simulink model "Missile_Step_Impulse"  (R2018b)
settings: Solver=ode4  StartTime=0.0  StopTime=7  FixedStep=Step_Size  RelTol=1e-3
InitFcn:
  | clc ;
  | clear all ;
  | close all ;
  | Missile_Data ;
  | Sim_Parameters ;
values from neighbouring files (symbols this model uses):
  ALT = [0.0 1000 2000 3000 4000]    [Sim_Parameters.m]
  Init_Rate = [ 0.0, 0.0, 0.0 ] * UNIT_DEG2RAD    [Sim_Parameters.m]
  Init_Vel = [ 238.0, 0.0, 0.0 ]    [Sim_Parameters.m]
  SOS_Table = [340.268 336.408 332.504  328.553 324.554]    [Sim_Parameters.m]
  UNIT_GRAV = 9.81    [Sim_Parameters.m]
undefined symbols (not defined in the file or in its folder): Alt_Trim, D, Mass, S, Tbl_ALPHAT, Tbl_CL_ALPHAT, Tbl_CL_DEL_R, Tbl_CL_P, Tbl_CM_0, Tbl_CM_DEL_P, Tbl_CM_PHIT, Tbl_CM_Q, Tbl_CN_DEL_Y, Tbl_CN_PHIT, Tbl_CN_R, Tbl_CX_0, Tbl_CX_ALPHAT, Tbl_CX_DEL_EFF, Tbl_CY_DEL_Y, Tbl_CY_PHIT, Tbl_CZ_0, Tbl_CZ_DEL_P, Tbl_CZ_PHIT, Tbl_MACH, XCG, XREF
libraries: simulink_extras x13, aerolibtransform2 x4, UAS_Model_library x4, aerolibasang x3, dspsrcs4 x3, shared6dofsys x1, sharedutil x1, shared6dof x1
settings Model: Creator=e803534  LastModifiedBy=auten
settings OptimizationCC: LifeSpan=inf
settings DebuggingCC: LibraryContextMissingDiagnostic=none  SFUnexpectedBacktrackingDiag=warning  SFNoUnconditionalDefaultTransitionDiag=warning  SFExecutionAtInitializationDiag=none
settings SFSimCC: SimUseLocalCustomCode=off
settings RTWCC: RTWUseLocalCustomCode=off
settings CodeAppCC: StateflowObjectComments=on
settings GRTTargetCC: TargetLangStandard=C89/C90 (ANSI)  GeneratePreprocessorConditionals=Disable all
settings ConfigComp: CovMetricSettings=dw  CovHtmlReporting=on  CovSaveCumulativeToWorkspaceVar=on  CovSaveSingleToWorkspaceVar=on  CovExternalEMLEnable=off

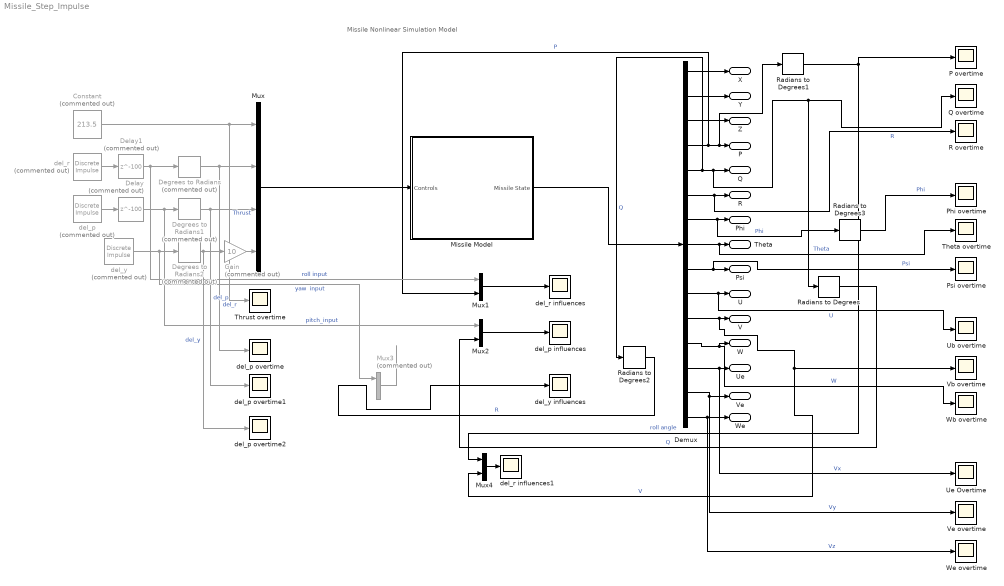
== system Missile_Step_Impulse ==
  note: Missile Nonlinear Simulation Model
  Constant : Constant  Commented=on  Value=213.5  VectorParams1D=off  SampleTime=-1
  Degrees to Radians : simulink_extras/Transformations/Degrees to Radians  Commented=on
  Degrees to Radians1 : simulink_extras/Transformations/Degrees to Radians  Commented=on
  Degrees to Radians2 : simulink_extras/Transformations/Degrees to Radians  Commented=on
  Delay : Delay  Commented=on  DelayLength=100
  Delay1 : Delay  Commented=on  DelayLength=100
  Demux : Demux  Outputs=15
  Gain : Gain  Commented=on  Gain=10
  Missile Model : Subsystem
  Mux : Mux
  Mux1 : Mux  Inputs=2
  Mux2 : Mux  Inputs=2
  Mux3 : Mux  Commented=on  Inputs=3
  Mux4 : Mux  Inputs=2
  P overtime : Scope
  Phi overtime : Scope
  Psi overtime : Scope
  Q overtime : Scope
  R overtime : Scope
  Radians to Degrees{,1..3} (4 alike) : simulink_extras/Transformations/Radians to Degrees
  Theta overtime : Scope
  Thrust overtime : Scope
  Ub overtime : Scope
  Ue Overtime : Scope
  Vb overtime : Scope
  Ve overtime : Scope
  Wb overtime : Scope
  We overtime : Scope
  del_p : dspsrcs4/Discrete  Impulse  Commented=on  Delay=1  SampleTime=0.1  FrameSample=1  OutputFrames=off  dataType=double  isSigned=on  wordLen=16  udDataType=sfix(16)  fracBitsMode=Best precision  numFracBits=15  OutDataTypeStr=double  LastOutDataTypeStr=double
  del_p influences : Scope
  del_p overtime : Scope
  del_p overtime1 : Scope
  del_p overtime2 : Scope
  "del_r " : dspsrcs4/Discrete  Impulse  Commented=on  Delay=1  SampleTime=0.1  FrameSample=1  OutputFrames=off  dataType=double  isSigned=on  wordLen=16  udDataType=sfix(16)  fracBitsMode=Best precision  numFracBits=15  OutDataTypeStr=double  LastOutDataTypeStr=double
  del_r influences : Scope
  del_r influences1 : Scope
  del_y : dspsrcs4/Discrete  Impulse  Commented=on  Delay=1  SampleTime=0.001  FrameSample=1  OutputFrames=off  dataType=double  isSigned=on  wordLen=16  udDataType=sfix(16)  fracBitsMode=Best precision  numFracBits=15  OutDataTypeStr=double  LastOutDataTypeStr=double
  del_y influences : Scope
  X : Outport
  Y : Outport  Port=2
  Z : Outport  Port=3
  P : Outport  Port=4
  Q : Outport  Port=5
  R : Outport  Port=6
  Phi : Outport  Port=7
  Theta : Outport  Port=8
  Psi : Outport  Port=9
  U : Outport  Port=10
  V : Outport  Port=11
  W : Outport  Port=12
  Ue : Outport  Port=13
  Ve : Outport  Port=14
  We : Outport  Port=15
  wires:
  Mux/1 -> Missile Model/1(Controls)
  Demux/11 -> Mux4/2, Vb overtime/1, V/1  "V"
  Demux/4 -> Mux1/2, Radians to Degrees1/1, P/1  "P"
  Demux/10 -> Ub overtime/1, U/1  "U"
  Demux/6 -> R overtime/1, R/1  "R"
  Demux/9 -> Psi overtime/1, Psi/1  "Psi"
  Demux/3 -> Z/1
  Demux/2 -> Y/1
  Demux/12 -> Wb overtime/1, W/1  "W"
  Demux/5 -> Radians to Degrees2/1, Radians to Degrees/1, Q overtime/1, Q/1  "Q"
  Demux/1 -> X/1
  Demux/7 -> Radians to Degrees3/1, Phi/1  "Phi"
  Missile Model/1(Missile State) -> Demux/1
  Degrees to Radians/1 -> del_p overtime/1, Mux/2  "del_r"
  Degrees to Radians1/1 -> Mux/3, del_p overtime1/1  "del_p"
  Degrees to Radians2/1 -> Gain/1, del_p overtime2/1  "del_y"
  Demux/15 -> We overtime/1, We/1  "Vz"
  Demux/14 -> Ve/1, Ve overtime/1  "Vy"
  Demux/13 -> Ue Overtime/1, Ue/1  "Vx"
  Demux/8 -> Theta overtime/1, Theta/1  "Theta"
  "del_r "/1 -> Delay1/1
  del_p/1 -> Delay/1
  Delay/1 -> Degrees to Radians1/1, Mux2/1  "pitch_input"
  Constant/1 -> Thrust overtime/1, Mux/1  "Thrust"
  del_y/1 -> Mux3/1, Degrees to Radians2/1  "yaw  input"
  Delay1/1 -> Mux1/1, Degrees to Radians/1  "roll input"
  Mux1/1 -> del_r influences/1
  Mux2/1 -> del_p influences/1
  Mux3/1 -> ?
  Radians to Degrees1/1 -> P overtime/1, Mux4/1  "roll angle"
  Mux4/1 -> del_r influences1/1
  Radians to Degrees/1 -> Mux2/2  "Q"
  Radians to Degrees2/1 -> del_y influences/1  "R"
  Gain/1 -> Mux/4
  Radians to Degrees3/1 -> Phi overtime/1  "Phi"

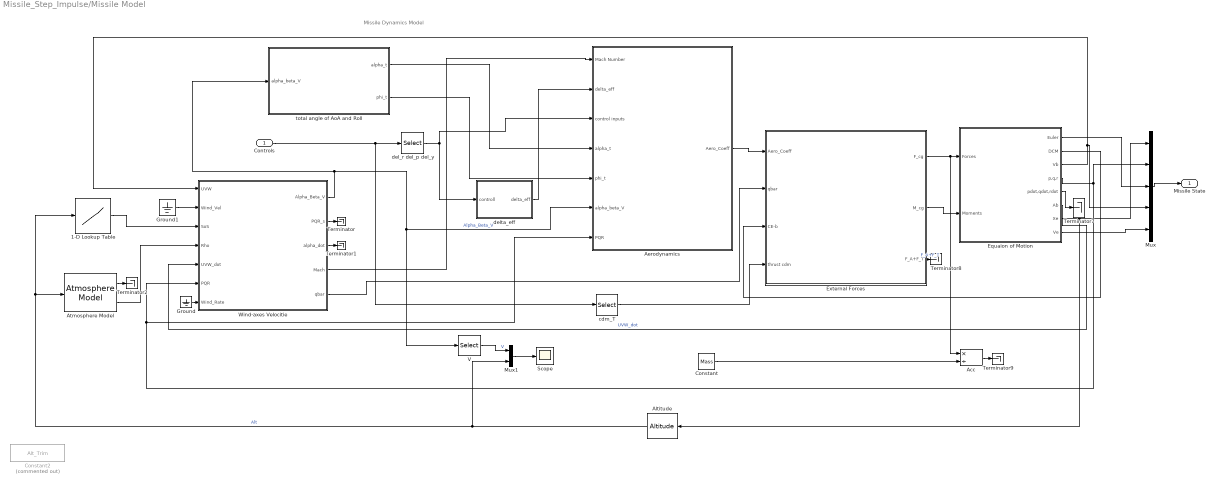
== system Missile_Step_Impulse/Missile Model ==
  note: Missile Dynamics Model
  Controls : Inport
  1-D Lookup Table : Lookup_n-D  NumberOfTableDimensions=1  BreakpointsForDimension1=ALT  Table=SOS_Table  InternalRulePriority=Speed  RndMeth=Simplest  InputSameDT=on
  Acc : Product  Inputs=*/  RndMeth=Zero
  Aerodynamics : Subsystem
  Altitude : UAS_Model_library/Equations of Motion/Altitude  SystemSampleTime=-1
  Atmosphere Model : UAS_Model_library/Envrionment/Atmosphere Model  SystemSampleTime=-1
  Constant : Constant  Value=Mass
  Constant2 : Constant  Commented=on  Value=Alt_Trim
  Equaion of Motion : Subsystem
  External Forces : Subsystem
  Ground : Ground
  Ground1 : Ground
  Mux : Mux  Inputs=5
  Mux1 : Mux  Inputs=2
  Scope : Scope
  Terminator{,1..2,7..9} (6 alike) : Terminator
  V : Selector  InputPortWidth=3  IndexOptions=Index vector (dialog)  Indices=[3]  OutputSizes=1
  Wind-axes Velocitie : Subsystem  AncestorBlock=UAS_Model_library/External Forces/Aerodynamics/Wind-axes Velocitie
  cdm_T : Selector  InputPortWidth=4  IndexOptions=Index vector (dialog)  Indices=[1]  OutputSizes=1
  del_r del_p del_y : Selector  InputPortWidth=4  IndexOptions=Index vector (dialog)  Indices=[2 3 4]  OutputSizes=1
  delta_eff : Subsystem
  total angle of AoA and Roll : Subsystem
  Missile State : Outport
  wires:
  Atmosphere Model/2 -> Wind-axes Velocitie/4(Rho)
  Controls/1 -> del_r del_p del_y/1, cdm_T/1
  External Forces/1(F_cg) -> Acc/1, Equaion of Motion/1(Forces)
  External Forces/2(M_cg) -> Equaion of Motion/2(Moments)
  Constant/1 -> Acc/2
  Mux/1 -> Missile State/1
  Equaion of Motion/3(Vb) -> Mux/4, Wind-axes Velocitie/1(UVW)
  Equaion of Motion/4(p,q,r) -> Aerodynamics/7(PQR), Wind-axes Velocitie/6(PQR), Mux/2
  Acc/1 -> Terminator9/1
  Equaion of Motion/1(Euler) -> Mux/3
  Equaion of Motion/2(DCM) -> External Forces/3(CE-b)
  Altitude/1 -> 1-D Lookup Table/1, Atmosphere Model/1, Mux1/2  "Alt"
  Wind-axes Velocitie/1(Alpha_Beta_V) -> V/1, Aerodynamics/6(alpha_beta_V), total angle of AoA and Roll/1(alpha_beta_V)  "Alpha_Beta_V"
  Wind-axes Velocitie/2(PQR_s) -> Terminator/1
  Wind-axes Velocitie/3(alpha_dot) -> Terminator1/1
  total angle of AoA and Roll/2(phi_t) -> Aerodynamics/5(phi_t)
  Aerodynamics/1(Aero_Coeff) -> External Forces/1(Aero_Coeff)
  total angle of AoA and Roll/1(alpha_t) -> Aerodynamics/4(alpha_t)
  delta_eff/1(delta_eff) -> Aerodynamics/2(delta_eff)
  cdm_T/1 -> External Forces/4(thrust cdm)
  Wind-axes Velocitie/4(Mach) -> Aerodynamics/1(Mach Number)
  Wind-axes Velocitie/5(qbar) -> External Forces/2(qbar)
  del_r del_p del_y/1 -> Aerodynamics/3(control inputs), delta_eff/1(controll)
  Atmosphere Model/1 -> Terminator2/1
  1-D Lookup Table/1 -> Wind-axes Velocitie/3(SoS)
  Ground1/1 -> Wind-axes Velocitie/2(Wind_Vel)
  Equaion of Motion/5(pdot,qdot,rdot) -> Terminator7/1
  Equaion of Motion/6(Ab) -> Wind-axes Velocitie/5(UVW_dot)  "UVW_dot"
  Ground/1 -> Wind-axes Velocitie/7(Wind_Rate)
  External Forces/3(F_A+F_T) -> Terminator8/1  "F_A+F_T"
  Equaion of Motion/7(Xe) -> Altitude/1, Mux/1
  Equaion of Motion/8(Ve) -> Mux/5
  V/1 -> Mux1/1  "V"
  Mux1/1 -> Scope/1

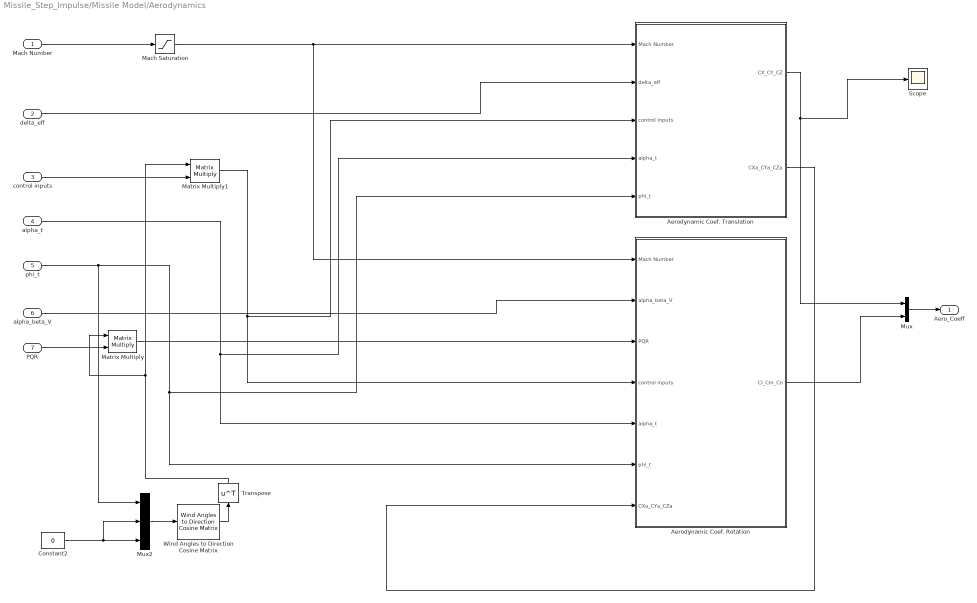
== system Missile_Step_Impulse/Missile Model/Aerodynamics ==
  Mach Number : Inport
  delta_eff : Inport  Port=2
  control inputs : Inport  Port=3
  alpha_t : Inport  Port=4
  phi_t : Inport  Port=5
  alpha_beta_V : Inport  Port=6
  PQR : Inport  Port=7
  Aerodynamic Coef. Rotation : Subsystem
  Aerodynamic Coef. Translation : Subsystem
  Constant2 : Constant  Value=0
  Mach Saturation : Saturate  UpperLimit=0.7  LowerLimit=0.2
  Matrix Multiply : Product  Multiplication=Matrix(*)
  Matrix Multiply1 : Product  Multiplication=Matrix(*)
  Mux : Mux  Inputs=2
  Mux2 : Mux  Inputs=3
  Scope : Scope
  Transpose : Math  Operator=transpose  SaturateOnIntegerOverflow=on
  Wind Angles to Direction Cosine Matrix : aerolibtransform2/Wind Angles to  Direction Cosine Matrix
      settings: SourceProductName=Aerospace Blockset  SourceProductBaseCode=AE
  Aero_Coeff : Outport
  wires:
  Aerodynamic Coef. Translation/2(CXa_CYa_CZa) -> Aerodynamic Coef. Rotation/7(CXa_CYa_CZa)
  Mach Number/1 -> Mach Saturation/1
  delta_eff/1 -> Aerodynamic Coef. Translation/2(delta_eff)
  Matrix Multiply1/1 -> Aerodynamic Coef. Rotation/4(control inputs), Aerodynamic Coef. Translation/3(control inputs)
  alpha_beta_V/1 -> Aerodynamic Coef. Rotation/2(alpha_beta_V)
  Matrix Multiply/1 -> Aerodynamic Coef. Rotation/3(PQR)
  Aerodynamic Coef. Translation/1(CX_CY_CZ) -> Scope/1, Mux/1
  Aerodynamic Coef. Rotation/1(Cl_Cm_Cn) -> Mux/2
  Mux/1 -> Aero_Coeff/1
  alpha_t/1 -> Aerodynamic Coef. Rotation/5(alpha_t), Aerodynamic Coef. Translation/4(alpha_t)
  phi_t/1 -> Mux2/1, Aerodynamic Coef. Translation/5(phi_t), Aerodynamic Coef. Rotation/6(phi_t)
  Mux2/1 -> Wind Angles to Direction Cosine Matrix/1
  Constant2/1 -> Mux2/2, Mux2/3
  control inputs/1 -> Matrix Multiply1/2
  Wind Angles to Direction Cosine Matrix/1 -> Transpose/1
  PQR/1 -> Matrix Multiply/2
  Transpose/1 -> Matrix Multiply/1, Matrix Multiply1/1
  Mach Saturation/1 -> Aerodynamic Coef. Rotation/1(Mach Number), Aerodynamic Coef. Translation/1(Mach Number)

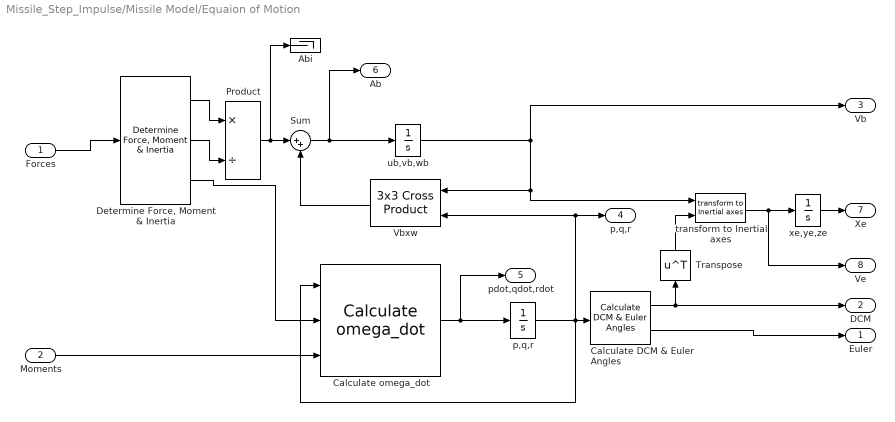
== system Missile_Step_Impulse/Missile Model/Equaion of Motion ==
  Forces : Inport  Unit=N  PortDimensions=3
  Moments : Inport  Port=2  Unit=N*m  PortDimensions=3
  Abi : Terminator
  Calculate DCM & Euler Angles : UAS_Model_library/Equations of Motion/Calculate DCM & Euler Angles  SystemSampleTime=-1
      link override phi theta psi: InitialCondition=[10*pi/180 0 0]
  Calculate omega_dot : shared6dofsys/Calculate omega_dot  aMode=aMode
      settings: SourceProductName=Aerospace Blockset  SourceProductBaseCode=AE
  "Determine Force, Moment & Inertia" : UAS_Model_library/Equations of Motion/Determine Force, Moment & Inertia  SystemSampleTime=-1
  Product : Product  Inputs=*/  SaturateOnIntegerOverflow=on  OutDataTypeStr=Inherit: Same as first input
  Sum : Sum  Inputs=|++  SaturateOnIntegerOverflow=on
  Transpose : Math  Operator=transpose  SaturateOnIntegerOverflow=on
  Vbxw : sharedutil/3x3 Cross Product  aMode=aMode
      settings: SourceProductBaseCode=AE
  "p,q,r " : Integrator  InitialCondition=Init_Rate
  "transform to Inertial axes " : shared6dof/6DOF (Euler Angles)/transform to Inertial axes   SystemSampleTime=-1
      settings: SourceProductName=Aerospace Blockset  SourceProductBaseCode=AE
  ub,vb,wb : Integrator  InitialCondition=Init_Vel
  xe,ye,ze : Integrator  InitialCondition=[0 0 -2000]
  Euler : Outport  Unit=rad
  DCM : Outport  Port=2  Unit=1
  Vb : Outport  Port=3  Unit=m/s
  p,q,r : Outport  Port=4  Unit=rad/s
  pdot,qdot,rdot : Outport  Port=5  Unit=rad/s^2
  Ab : Outport  Port=6  Unit=m/s^2
  Xe : Outport  Port=7  Unit=m/s
  Ve : Outport  Port=8  Unit=m/s
  wires:
  "transform to Inertial axes "/1 -> Ve/1, xe,ye,ze/1
  Calculate omega_dot/1 -> pdot,qdot,rdot/1, "p,q,r "/1
  Sum/1 -> ub,vb,wb/1, Ab/1
  Vbxw/1 -> Sum/2
  Product/1 -> Sum/1, Abi/1
  "p,q,r "/1 -> Calculate DCM & Euler Angles/1, Calculate omega_dot/1, p,q,r/1, Vbxw/2
  Forces/1 -> "Determine Force, Moment & Inertia"/1
  ub,vb,wb/1 -> Vb/1, "transform to Inertial axes "/1, Vbxw/1
  "Determine Force, Moment & Inertia"/2 -> Product/2
  Moments/1 -> Calculate omega_dot/3
  Calculate DCM & Euler Angles/2 -> Euler/1
  Calculate DCM & Euler Angles/1 -> Transpose/1, DCM/1
  "Determine Force, Moment & Inertia"/3 -> Calculate omega_dot/2
  Transpose/1 -> "transform to Inertial axes "/2
  "Determine Force, Moment & Inertia"/1 -> Product/1
  xe,ye,ze/1 -> Xe/1

== system Missile_Step_Impulse/Missile Model/External Forces ==
  Aero_Coeff : Inport
  qbar : Inport  Port=2
  CE-b : Inport  Port=3
  thrust cdm : Inport  Port=4
  Aerodynamic Force & Moment : Subsystem  AncestorBlock=UAS_Model_library/External Forces/Aerodynamics/Aerodynamic Force & Moment
  Propulsive Force & Moment : Subsystem  AncestorBlock=UAS_Model_library/External Forces/Propulsive/Propulsive Force & Moment
  Sum of Aerodynamic and Propulsion Forces : Sum
  Total Force & Moment : Subsystem  AncestorBlock=UAS_Model_library/External Forces/Total Force & Moment
  F_cg : Outport
  M_cg : Outport  Port=2
  F_A+F_T : Outport  Port=3
  wires:
  Total Force & Moment/2(M_cg) -> M_cg/1
  Aerodynamic Force & Moment/2(M_aero) -> Total Force & Moment/2(M_aero)
  Propulsive Force & Moment/2(M_prop) -> Total Force & Moment/4(M_prop)
  Total Force & Moment/1(F_cg) -> F_cg/1
  Aerodynamic Force & Moment/1(F_aero) -> Sum of Aerodynamic and Propulsion Forces/1, Total Force & Moment/1(F_aero)
  Propulsive Force & Moment/1(F_prop) -> Sum of Aerodynamic and Propulsion Forces/2, Total Force & Moment/3(F_prop)
  qbar/1 -> Aerodynamic Force & Moment/2(qbar)
  Aero_Coeff/1 -> Aerodynamic Force & Moment/1(Aero_Coeff)
  Sum of Aerodynamic and Propulsion Forces/1 -> F_A+F_T/1
  CE-b/1 -> Total Force & Moment/5("cE-B ")
  thrust cdm/1 -> Propulsive Force & Moment/1(Controls)

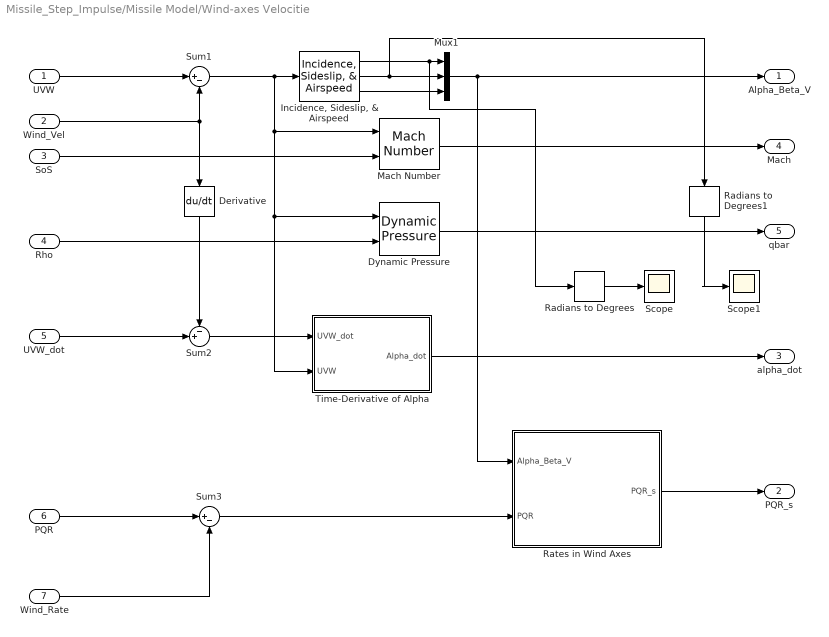
== system Missile_Step_Impulse/Missile Model/Wind-axes Velocitie ==
  UVW : Inport
  Wind_Vel : Inport  Port=2
  SoS : Inport  Port=3
  Rho : Inport  Port=4
  UVW_dot : Inport  Port=5
  PQR : Inport  Port=6
  Wind_Rate : Inport  Port=7
  Derivative : Derivative
  Dynamic Pressure : aerolibasang/Dynamic Pressure
  "Incidence, Sideslip, & Airspeed" : aerolibasang/Incidence, Sideslip, & Airspeed
      settings: SourceProductName=Aerospace Blockset
  Mach Number : aerolibasang/Mach Number
      settings: SourceProductName=Aerospace Blockset  SourceProductBaseCode=AE
  Mux1 : Mux  Inputs=3
  Radians to Degrees : simulink_extras/Transformations/Radians to Degrees
  Radians to Degrees1 : simulink_extras/Transformations/Radians to Degrees
  Rates in Wind Axes : Subsystem
  Scope : Scope
  Scope1 : Scope
  Sum1 : Sum  Inputs=|+-  SaturateOnIntegerOverflow=on  InputSameDT=on  OutDataTypeStr=Inherit: Same as first input
  Sum2 : Sum  Inputs=-+|  SaturateOnIntegerOverflow=on  InputSameDT=on  OutDataTypeStr=Inherit: Same as first input
  Sum3 : Sum  Inputs=|+-  SaturateOnIntegerOverflow=on  InputSameDT=on  OutDataTypeStr=Inherit: Same as first input
  Time-Derivative of Alpha : Subsystem
  Alpha_Beta_V : Outport
  PQR_s : Outport  Port=2
  alpha_dot : Outport  Port=3
  Mach : Outport  Port=4
  qbar : Outport  Port=5
  wires:
  Wind_Rate/1 -> Sum3/2
  PQR/1 -> Sum3/1
  Sum3/1 -> Rates in Wind Axes/2(PQR)
  Rates in Wind Axes/1(PQR_s) -> PQR_s/1
  "Incidence, Sideslip, & Airspeed"/3 -> Mux1/3
  "Incidence, Sideslip, & Airspeed"/2 -> Radians to Degrees1/1, Mux1/2
  "Incidence, Sideslip, & Airspeed"/1 -> Radians to Degrees/1, Mux1/1
  Sum1/1 -> "Incidence, Sideslip, & Airspeed"/1, Mach Number/1, Dynamic Pressure/1, Time-Derivative of Alpha/2(UVW)
  Mux1/1 -> Alpha_Beta_V/1, Rates in Wind Axes/1(Alpha_Beta_V)
  UVW/1 -> Sum1/1
  Wind_Vel/1 -> Derivative/1, Sum1/2
  Mach Number/1 -> Mach/1
  SoS/1 -> Mach Number/2
  Rho/1 -> Dynamic Pressure/2
  Dynamic Pressure/1 -> qbar/1
  Time-Derivative of Alpha/1(Alpha_dot) -> alpha_dot/1
  UVW_dot/1 -> Sum2/2
  Sum2/1 -> Time-Derivative of Alpha/1(UVW_dot)
  Derivative/1 -> Sum2/1
  Radians to Degrees/1 -> Scope/1
  Radians to Degrees1/1 -> Scope1/1

== system Missile_Step_Impulse/Missile Model/delta_eff ==
  controll : Inport
  Abs : Abs
  Abs1 : Abs
  Constant : Constant  Value=2
  Divide : Product  Inputs=*/  SaturateOnIntegerOverflow=on  RndMeth=Zero
  Selector : Selector  InputPortWidth=3  IndexOptions=Index vector (dialog)  Indices=[3]  OutputSizes=1
  Selector1 : Selector  InputPortWidth=3  IndexOptions=Index vector (dialog)  Indices=[2]  OutputSizes=1
  Sum : Sum  Inputs=|++
  delta_eff : Outport
  wires:
  Selector1/1 -> Abs1/1
  Sum/1 -> Divide/1
  Constant/1 -> Divide/2
  Divide/1 -> delta_eff/1
  controll/1 -> Selector/1, Selector1/1
  Selector/1 -> Abs/1
  Abs/1 -> Sum/1
  Abs1/1 -> Sum/2

== system Missile_Step_Impulse/Missile Model/total angle of AoA and Roll ==
  alpha_beta_V : Inport
  Asin : Trigonometry  Operator=acos
  Atan2 : Trigonometry  Operator=atan2
  Cos : Trigonometry  Operator=cos
  Cos1 : Trigonometry  Operator=cos
  Multiply : Product
  Selector : Selector  InputPortWidth=3  IndexOptions=Index vector (dialog)  Indices=[1]  OutputSizes=1
  Selector1 : Selector  InputPortWidth=3  IndexOptions=Index vector (dialog)  Indices=[2]  OutputSizes=1
  Sin : Trigonometry
  Tan : Trigonometry  Operator=tan
  alpha_t : Outport
  phi_t : Outport  Port=2
  wires:
  Sin/1 -> Atan2/2
  Tan/1 -> Atan2/1
  Selector/1 -> Sin/1, Cos/1
  Selector1/1 -> Tan/1, Cos1/1
  Cos1/1 -> Multiply/2
  Multiply/1 -> Asin/1
  Cos/1 -> Multiply/1
  Atan2/1 -> phi_t/1
  Asin/1 -> alpha_t/1
  alpha_beta_V/1 -> Selector1/1, Selector/1

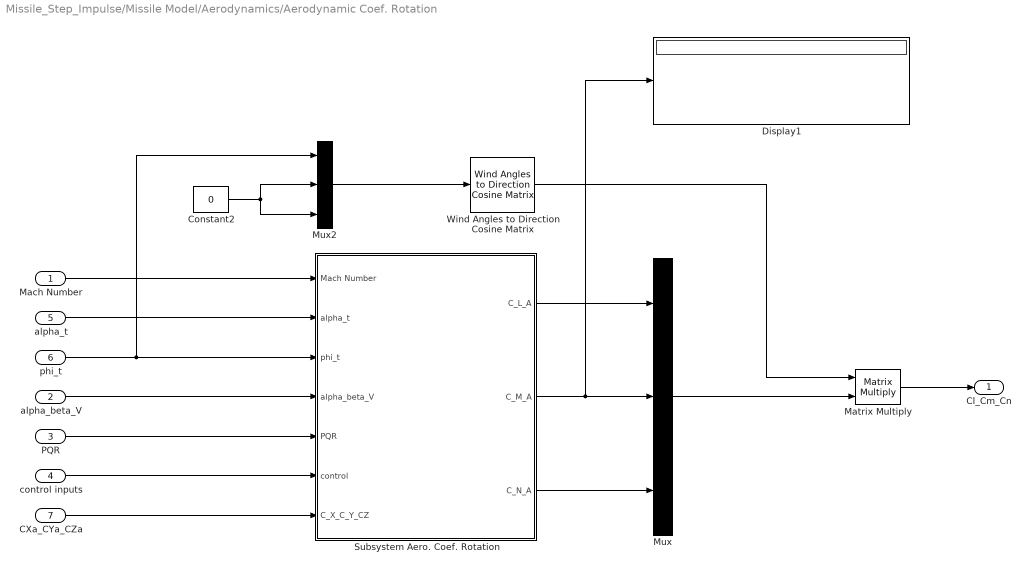
== system Missile_Step_Impulse/Missile Model/Aerodynamics/Aerodynamic Coef. Rotation ==
  Mach Number : Inport
  alpha_beta_V : Inport  Port=2
  PQR : Inport  Port=3
  control inputs : Inport  Port=4
  alpha_t : Inport  Port=5
  phi_t : Inport  Port=6
  CXa_CYa_CZa : Inport  Port=7
  Constant2 : Constant  Value=0
  Display1 : Display
  Matrix Multiply : Product  Multiplication=Matrix(*)
  Mux : Mux  Inputs=3
  Mux2 : Mux  Inputs=3
  Subsystem Aero. Coef. Rotation : Subsystem
  Wind Angles to Direction Cosine Matrix : aerolibtransform2/Wind Angles to  Direction Cosine Matrix
      settings: SourceProductName=Aerospace Blockset  SourceProductBaseCode=AE
  Cl_Cm_Cn : Outport
  wires:
  Mux/1 -> Matrix Multiply/2
  Matrix Multiply/1 -> Cl_Cm_Cn/1
  Mach Number/1 -> Subsystem Aero. Coef. Rotation/1(Mach Number)
  alpha_beta_V/1 -> Subsystem Aero. Coef. Rotation/4(alpha_beta_V)
  PQR/1 -> Subsystem Aero. Coef. Rotation/5(PQR)
  control inputs/1 -> Subsystem Aero. Coef. Rotation/6(control)
  alpha_t/1 -> Subsystem Aero. Coef. Rotation/2(alpha_t)
  phi_t/1 -> Mux2/1, Subsystem Aero. Coef. Rotation/3(phi_t)
  CXa_CYa_CZa/1 -> Subsystem Aero. Coef. Rotation/7(C_X_C_Y_CZ)
  Mux2/1 -> Wind Angles to Direction Cosine Matrix/1
  Constant2/1 -> Mux2/2, Mux2/3
  Wind Angles to Direction Cosine Matrix/1 -> Matrix Multiply/1
  Subsystem Aero. Coef. Rotation/1(C_L_A) -> Mux/1
  Subsystem Aero. Coef. Rotation/2(C_M_A) -> Display1/1, Mux/2
  Subsystem Aero. Coef. Rotation/3(C_N_A) -> Mux/3

== system Missile_Step_Impulse/Missile Model/Aerodynamics/Aerodynamic Coef. Translation ==
  Mach Number : Inport
  delta_eff : Inport  Port=2
  control inputs : Inport  Port=3
  alpha_t : Inport  Port=4
  phi_t : Inport  Port=5
  Constant2 : Constant  Value=0
  Matrix Multiply : Product  Multiplication=Matrix(*)
  Mux : Mux  Inputs=3
  Mux2 : Mux  Inputs=3
  Scope : Scope
  Subsystem Aero. Coef. Translation : Subsystem
  Transpose : Math  Commented=on  Operator=transpose  SaturateOnIntegerOverflow=on
  Wind Angles to Direction Cosine Matrix : aerolibtransform2/Wind Angles to  Direction Cosine Matrix
      settings: SourceProductName=Aerospace Blockset  SourceProductBaseCode=AE
  CX_CY_CZ : Outport
  CXa_CYa_CZa : Outport  Port=2
  wires:
  Mux/1 -> Matrix Multiply/2, CXa_CYa_CZa/1
  Matrix Multiply/1 -> CX_CY_CZ/1
  Mux2/1 -> Wind Angles to Direction Cosine Matrix/1
  phi_t/1 -> Mux2/1, Subsystem Aero. Coef. Translation/5(phi_t)
  Constant2/1 -> Mux2/2, Mux2/3
  Mach Number/1 -> Subsystem Aero. Coef. Translation/1(Mach number)
  control inputs/1 -> Subsystem Aero. Coef. Translation/4(control)
  alpha_t/1 -> Subsystem Aero. Coef. Translation/2(alpha_t)
  delta_eff/1 -> Subsystem Aero. Coef. Translation/3(delta_eff)
  Subsystem Aero. Coef. Translation/1(C_X_A) -> Scope/1, Mux/1
  Subsystem Aero. Coef. Translation/2(C_Y_A) -> Mux/2
  Subsystem Aero. Coef. Translation/3(C_Z_A) -> Mux/3
  Wind Angles to Direction Cosine Matrix/1 -> Matrix Multiply/1

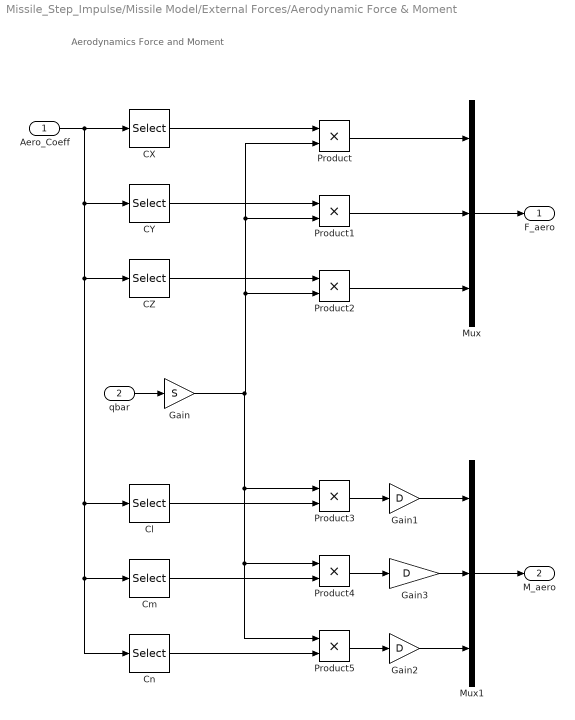
== system Missile_Step_Impulse/Missile Model/External Forces/Aerodynamic Force & Moment ==
  note: Aerodynamics Force and Moment
  Aero_Coeff : Inport
  qbar : Inport  Port=2
  CX : Selector  InputPortWidth=6  IndexOptions=Index vector (dialog)  Indices=[1]  OutputSizes=1
  CY : Selector  InputPortWidth=6  IndexOptions=Index vector (dialog)  Indices=[2]  OutputSizes=1
  CZ : Selector  InputPortWidth=6  IndexOptions=Index vector (dialog)  Indices=[3]  OutputSizes=1
  Cl : Selector  InputPortWidth=6  IndexOptions=Index vector (dialog)  Indices=[4]  OutputSizes=1
  Cm : Selector  InputPortWidth=6  IndexOptions=Index vector (dialog)  Indices=[5]  OutputSizes=1
  Cn : Selector  InputPortWidth=6  IndexOptions=Index vector (dialog)  Indices=[6]  OutputSizes=1
  Gain : Gain  Gain=S
  Gain1 : Gain  Gain=D
  Gain2 : Gain  Gain=D
  Gain3 : Gain  Gain=D
  Mux : Mux  Inputs=3
  Mux1 : Mux  Inputs=3
  Product{,1..5} (6 alike) : Product
  F_aero : Outport
  M_aero : Outport  Port=2
  wires:
  Gain3/1 -> Mux1/2
  Gain2/1 -> Mux1/3
  Gain1/1 -> Mux1/1
  Mux1/1 -> M_aero/1
  Product5/1 -> Gain2/1
  Product4/1 -> Gain3/1
  Product3/1 -> Gain1/1
  Cn/1 -> Product5/2
  Cm/1 -> Product4/2
  Cl/1 -> Product3/2
  Mux/1 -> F_aero/1
  Product2/1 -> Mux/3
  Product1/1 -> Mux/2
  Product/1 -> Mux/1
  CZ/1 -> Product2/1
  CY/1 -> Product1/1
  Gain/1 -> Product/2, Product1/2, Product2/2, Product3/1, Product4/1, Product5/1
  CX/1 -> Product/1
  qbar/1 -> Gain/1
  Aero_Coeff/1 -> CX/1, CY/1, CZ/1, Cm/1, Cn/1, Cl/1

== system Missile_Step_Impulse/Missile Model/External Forces/Propulsive Force & Moment ==
  note: Propulsive Force and Moment
  Controls : Inport
  Constant : Constant  Value=0
  Mux : Mux  Inputs=3
  Mux1 : Mux  Inputs=3
  F_prop : Outport
  M_prop : Outport  Port=2
  wires:
  Mux/1 -> F_prop/1
  Controls/1 -> Mux/1
  Constant/1 -> Mux/2, Mux1/1, Mux1/2, Mux1/3, Mux/3
  Mux1/1 -> M_prop/1

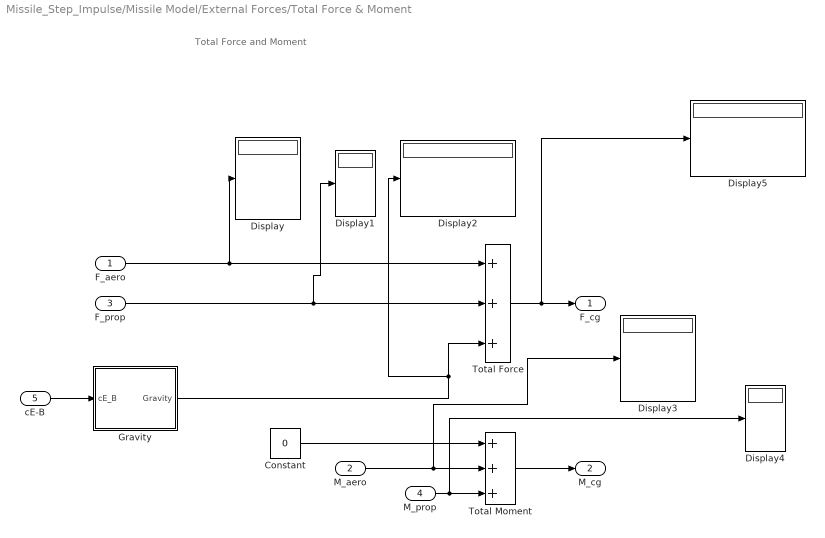
== system Missile_Step_Impulse/Missile Model/External Forces/Total Force & Moment ==
  note: Total Force and Moment
  F_aero : Inport  PortDimensions=3
  M_aero : Inport  Port=2  PortDimensions=3
  F_prop : Inport  Port=3  PortDimensions=3
  M_prop : Inport  Port=4  PortDimensions=3
  "cE-B " : Inport  Port=5
  Constant : Constant  Value=0
  Display{,1..5} (6 alike) : Display
  Gravity : Subsystem  AncestorBlock=UAS_Model_library/Envrionment/Gravity
  Total Force : Sum  Inputs=+++  SaturateOnIntegerOverflow=on  InputSameDT=on  OutDataTypeStr=Inherit: Same as first input
  Total Moment : Sum  Inputs=+++  SaturateOnIntegerOverflow=on  InputSameDT=on  OutDataTypeStr=Inherit: Same as first input
  F_cg : Outport
  M_cg : Outport  Port=2
  wires:
  Gravity/1(Gravity) -> Total Force/3, Display2/1
  Total Moment/1 -> M_cg/1
  M_prop/1 -> Display4/1, Total Moment/3
  F_prop/1 -> Display1/1, Total Force/2
  F_aero/1 -> Display/1, Total Force/1
  Constant/1 -> Total Moment/1
  M_aero/1 -> Display3/1, Total Moment/2
  "cE-B "/1 -> Gravity/1(cE_B)
  Total Force/1 -> Display5/1, F_cg/1

== system Missile_Step_Impulse/Missile Model/Wind-axes Velocitie/Rates in Wind Axes ==
  note: Rates in Wind Axes
  Alpha_Beta_V : Inport
  PQR : Inport  Port=2
  Alpha : Selector  InputPortWidth=3  IndexOptions=Index vector (dialog)  Indices=[1]  OutputSizes=1
  Beta_Ref : Constant  Value=0
  Direction Cosine Matrix Body to Wind : aerolibtransform2/Direction Cosine Matrix Body to Wind
      settings: SourceProductName=Aerospace Blockset  SourceProductBaseCode=AE
  Mux : Mux  Inputs=2
  transform to body axes : Product  Inputs=**  Multiplication=Matrix(*)  SaturateOnIntegerOverflow=on  InputSameDT=on  OutDataTypeStr=Inherit: Same as first input
  PQR_s : Outport
  wires:
  Beta_Ref/1 -> Mux/2
  Mux/1 -> Direction Cosine Matrix Body to Wind/1
  transform to body axes/1 -> PQR_s/1
  PQR/1 -> transform to body axes/2
  Direction Cosine Matrix Body to Wind/1 -> transform to body axes/1  "cB_W"
  Alpha/1 -> Mux/1
  Alpha_Beta_V/1 -> Alpha/1

== system Missile_Step_Impulse/Missile Model/Wind-axes Velocitie/Time-Derivative of Alpha ==
  note: Time Derivative of Alpha
  UVW_dot : Inport
  UVW : Inport  Port=2
  Add : Sum  Inputs=-+
  Add1 : Sum
  Demux2 : Demux  Outputs=3
  Demux3 : Demux  Outputs=3
  Divide : Product  Inputs=*/
  Math Function2 : Math  Operator=square  SaturateOnIntegerOverflow=on
  Math Function3 : Math  Operator=square  SaturateOnIntegerOverflow=on
  Product3 : Product
  Product4 : Product
  Terminator2 : Terminator
  Terminator3 : Terminator
  Alpha_dot : Outport
  wires:
  Divide/1 -> Alpha_dot/1
  Add1/1 -> Divide/2
  Math Function3/1 -> Add1/2
  Math Function2/1 -> Add1/1
  Add/1 -> Divide/1
  Product3/1 -> Add/1
  Product4/1 -> Add/2
  Demux3/1 -> Product4/2, Math Function2/1
  Demux2/3 -> Product4/1
  Demux3/3 -> Product3/2, Math Function3/1
  Demux3/2 -> Terminator3/1
  UVW/1 -> Demux3/1
  Demux2/1 -> Product3/1
  Demux2/2 -> Terminator2/1
  UVW_dot/1 -> Demux2/1

== system Missile_Step_Impulse/Missile Model/Aerodynamics/Aerodynamic Coef. Rotation/Subsystem Aero. Coef. Rotation ==
  Mach Number : Inport
  alpha_t : Inport  Port=2
  phi_t : Inport  Port=3
  alpha_beta_V : Inport  Port=4
  PQR : Inport  Port=5
  control : Inport  Port=6
  C_X_C_Y_CZ : Inport  Port=7
  "Subsystem C_L_A " : Subsystem
  "Subsystem C_M_A " : Subsystem
  Subsystem C_N_A : Subsystem
  C_L_A : Outport
  C_M_A : Outport  Port=2
  C_N_A : Outport  Port=3
  wires:
  "Subsystem C_M_A "/1(C_M_A) -> C_M_A/1
  "Subsystem C_L_A "/1(C_L_A) -> C_L_A/1
  Subsystem C_N_A/1(C_N_A) -> C_N_A/1
  Mach Number/1 -> "Subsystem C_L_A "/1(Mach Number), "Subsystem C_M_A "/1(Mach Number), Subsystem C_N_A/1(Mach Number)
  alpha_t/1 -> Subsystem C_N_A/2(alpha_t), "Subsystem C_M_A "/2(alpha_t), "Subsystem C_L_A "/2(alpha_t)
  phi_t/1 -> Subsystem C_N_A/3(phi_t), "Subsystem C_M_A "/3(phi_t), "Subsystem C_L_A "/3(phi_t)
  alpha_beta_V/1 -> "Subsystem C_L_A "/4(alpha_beta_V), "Subsystem C_M_A "/4(alpha_beta_V), Subsystem C_N_A/4(alpha_beta_V)
  PQR/1 -> "Subsystem C_M_A "/5(PQR), "Subsystem C_L_A "/5(PQR), Subsystem C_N_A/5(PQR)
  control/1 -> "Subsystem C_M_A "/6(control), "Subsystem C_L_A "/6(control), Subsystem C_N_A/6(control)
  C_X_C_Y_CZ/1 -> "Subsystem C_M_A "/7(C_X_C_Y_C_Z), Subsystem C_N_A/7(C_X_C_Y_C_Z)

== system Missile_Step_Impulse/Missile Model/Aerodynamics/Aerodynamic Coef. Translation/Subsystem Aero. Coef. Translation ==
  Mach number : Inport
  alpha_t : Inport  Port=2
  delta_eff : Inport  Port=3
  control : Inport  Port=4
  phi_t : Inport  Port=5
  Subsystem C_X_A : Subsystem
  Subsystem C_Y_A : Subsystem
  Subsystem C_Z_A : Subsystem
  C_X_A : Outport
  C_Y_A : Outport  Port=2
  C_Z_A : Outport  Port=3
  wires:
  Subsystem C_X_A/1(C_X_A) -> C_X_A/1
  Subsystem C_Y_A/1(C_Y_A) -> C_Y_A/1
  Subsystem C_Z_A/1(C_Z_A) -> C_Z_A/1
  Mach number/1 -> Subsystem C_Z_A/1(Mach Number), Subsystem C_Y_A/1(Mach Number), Subsystem C_X_A/1(Mach Number)
  alpha_t/1 -> Subsystem C_Z_A/2(alpha_t), Subsystem C_Y_A/2(alpha_t), Subsystem C_X_A/2(alpha_t)
  delta_eff/1 -> Subsystem C_X_A/3(delta_eff)
  control/1 -> Subsystem C_Z_A/3(control), Subsystem C_Y_A/3(control)
  phi_t/1 -> Subsystem C_Z_A/4(phi_t), Subsystem C_Y_A/4(phi_t)

== system Missile_Step_Impulse/Missile Model/External Forces/Total Force & Moment/Gravity ==
  cE_B : Inport
  Constant : Constant  Value=0
  Constant1 : Constant  Value=Mass
  Display : Display
  Display1 : Display
  "Gravity vector in body frame " : Product  Multiplication=Matrix(*)  SaturateOnIntegerOverflow=on  InputSameDT=on  OutDataTypeStr=Inherit: Same as first input
  Mux1 : Mux  Inputs=3
  g : Gain  Gain=UNIT_GRAV
  Gravity : Outport
  wires:
  Constant1/1 -> g/1
  "Gravity vector in body frame "/1 -> Display/1, Gravity/1
  g/1 -> Mux1/3
  Mux1/1 -> "Gravity vector in body frame "/2
  cE_B/1 -> Display1/1, "Gravity vector in body frame "/1
  Constant/1 -> Mux1/1, Mux1/2

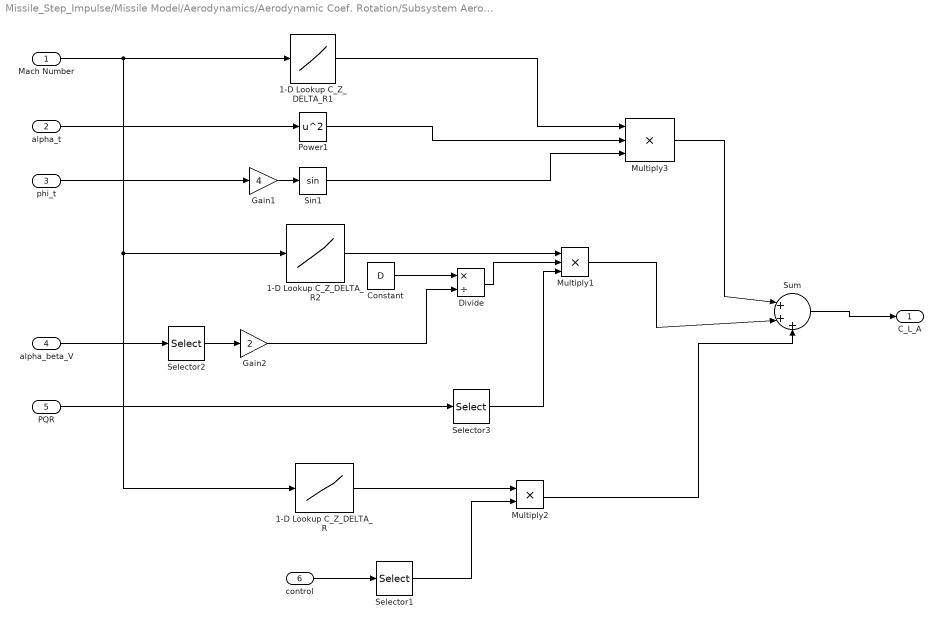
== system Missile_Step_Impulse/Missile Model/Aerodynamics/Aerodynamic Coef. Rotation/Subsystem Aero. Coef. Rotation/Subsystem C_L_A  ==
  Mach Number : Inport
  alpha_t : Inport  Port=2
  phi_t : Inport  Port=3
  alpha_beta_V : Inport  Port=4
  PQR : Inport  Port=5
  control : Inport  Port=6
  1-D Lookup C_Z_DELTA_R : Lookup_n-D  NumberOfTableDimensions=1  BreakpointsForDimension1=Tbl_MACH  Table=Tbl_CL_DEL_R  InternalRulePriority=Speed  RndMeth=Simplest  InputSameDT=on
  1-D Lookup C_Z_DELTA_R1 : Lookup_n-D  NumberOfTableDimensions=1  BreakpointsForDimension1=Tbl_MACH  Table=Tbl_CL_ALPHAT  InternalRulePriority=Speed  RndMeth=Simplest  InputSameDT=on
  1-D Lookup C_Z_DELTA_R2 : Lookup_n-D  NumberOfTableDimensions=1  BreakpointsForDimension1=Tbl_MACH  Table=Tbl_CL_P  InternalRulePriority=Speed  RndMeth=Simplest  InputSameDT=on
  Constant : Constant  Value=D
  Divide : Product  Inputs=*/
  Gain1 : Gain  Gain=4
  Gain2 : Gain  Gain=2
  Multiply1 : Product  Inputs=3
  Multiply2 : Product
  Multiply3 : Product  Inputs=3
  Power1 : Math  Operator=square  SaturateOnIntegerOverflow=on
  Selector1 : Selector  InputPortWidth=3  IndexOptions=Index vector (dialog)  Indices=[1]  OutputSizes=1
  Selector2 : Selector  InputPortWidth=3  IndexOptions=Index vector (dialog)  Indices=[3]  OutputSizes=1
  Selector3 : Selector  InputPortWidth=3  IndexOptions=Index vector (dialog)  Indices=[1]  OutputSizes=1
  Sin1 : Trigonometry
  Sum : Sum  Inputs=|+++
  C_L_A : Outport
  wires:
  1-D Lookup C_Z_DELTA_R1/1 -> Multiply3/1
  alpha_t/1 -> Power1/1
  Sum/1 -> C_L_A/1
  Mach Number/1 -> 1-D Lookup C_Z_DELTA_R/1, 1-D Lookup C_Z_DELTA_R2/1, 1-D Lookup C_Z_DELTA_R1/1
  1-D Lookup C_Z_DELTA_R2/1 -> Multiply1/1
  1-D Lookup C_Z_DELTA_R/1 -> Multiply2/1
  Multiply2/1 -> Sum/3
  Power1/1 -> Multiply3/2
  Sin1/1 -> Multiply3/3
  phi_t/1 -> Gain1/1
  Gain1/1 -> Sin1/1
  alpha_beta_V/1 -> Selector2/1
  Multiply3/1 -> Sum/1
  Multiply1/1 -> Sum/2
  Constant/1 -> Divide/1
  Selector2/1 -> Gain2/1
  Gain2/1 -> Divide/2
  Divide/1 -> Multiply1/2
  PQR/1 -> Selector3/1
  Selector3/1 -> Multiply1/3
  control/1 -> Selector1/1
  Selector1/1 -> Multiply2/2

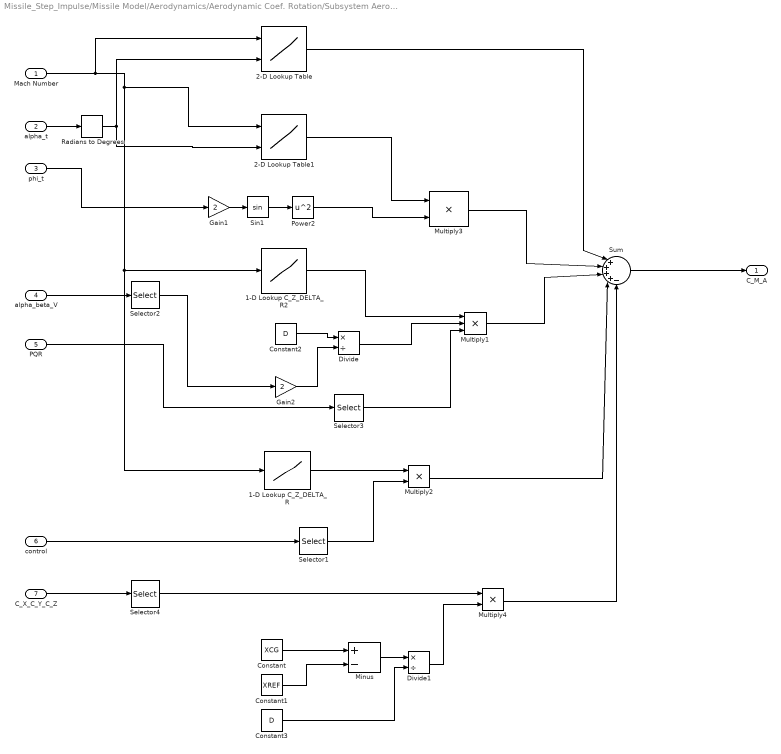
== system Missile_Step_Impulse/Missile Model/Aerodynamics/Aerodynamic Coef. Rotation/Subsystem Aero. Coef. Rotation/Subsystem C_M_A  ==
  Mach Number : Inport
  alpha_t : Inport  Port=2
  phi_t : Inport  Port=3
  alpha_beta_V : Inport  Port=4
  PQR : Inport  Port=5
  control : Inport  Port=6
  C_X_C_Y_C_Z : Inport  Port=7
  1-D Lookup C_Z_DELTA_R : Lookup_n-D  NumberOfTableDimensions=1  BreakpointsForDimension1=Tbl_MACH  Table=Tbl_CM_DEL_P  InternalRulePriority=Speed  RndMeth=Simplest  InputSameDT=on
  1-D Lookup C_Z_DELTA_R2 : Lookup_n-D  NumberOfTableDimensions=1  BreakpointsForDimension1=Tbl_MACH  Table=Tbl_CM_Q  DiagnosticForOutOfRangeInput=Warning  InternalRulePriority=Speed  RndMeth=Simplest  InputSameDT=on
  2-D Lookup Table : Lookup_n-D  BreakpointsForDimension1=Tbl_MACH  BreakpointsForDimension2=Tbl_ALPHAT  Table=Tbl_CM_0  DiagnosticForOutOfRangeInput=Warning  InternalRulePriority=Speed  RndMeth=Simplest  InputSameDT=on
  2-D Lookup Table1 : Lookup_n-D  BreakpointsForDimension1=Tbl_MACH  BreakpointsForDimension2=Tbl_ALPHAT  Table=Tbl_CM_PHIT  InternalRulePriority=Speed  RndMeth=Simplest  InputSameDT=on
  Constant : Constant  Value=XCG
  Constant1 : Constant  Value=XREF
  Constant2 : Constant  Value=D
  Constant3 : Constant  Value=D
  Divide : Product  Inputs=*/
  Divide1 : Product  Inputs=*/
  Gain1 : Gain  Gain=2
  Gain2 : Gain  Gain=2
  Minus : Sum  Inputs=+-
  Multiply1 : Product  Inputs=3
  Multiply2 : Product
  Multiply3 : Product
  Multiply4 : Product
  Power2 : Math  Operator=square  SaturateOnIntegerOverflow=on
  Radians to Degrees : simulink_extras/Transformations/Radians to Degrees
  Selector1 : Selector  InputPortWidth=3  IndexOptions=Index vector (dialog)  Indices=[2]  OutputSizes=1
  Selector2 : Selector  InputPortWidth=3  IndexOptions=Index vector (dialog)  Indices=[3]  OutputSizes=1
  Selector3 : Selector  InputPortWidth=3  IndexOptions=Index vector (dialog)  Indices=[2]  OutputSizes=1
  Selector4 : Selector  InputPortWidth=3  IndexOptions=Index vector (dialog)  Indices=[3]  OutputSizes=1
  Sin1 : Trigonometry
  Sum : Sum  Inputs=|++++-
  C_M_A : Outport
  wires:
  2-D Lookup Table/1 -> Sum/1
  Mach Number/1 -> 2-D Lookup Table/1, 2-D Lookup Table1/1, 1-D Lookup C_Z_DELTA_R/1, 1-D Lookup C_Z_DELTA_R2/1
  1-D Lookup C_Z_DELTA_R2/1 -> Multiply1/1
  1-D Lookup C_Z_DELTA_R/1 -> Multiply2/1
  Multiply2/1 -> Sum/4
  Sin1/1 -> Power2/1
  phi_t/1 -> Gain1/1
  Gain1/1 -> Sin1/1
  alpha_beta_V/1 -> Selector2/1
  Selector2/1 -> Gain2/1
  Gain2/1 -> Divide/2
  Divide/1 -> Multiply1/2
  PQR/1 -> Selector3/1
  Selector3/1 -> Multiply1/3
  control/1 -> Selector1/1
  Selector1/1 -> Multiply2/2
  2-D Lookup Table1/1 -> Multiply3/1
  Power2/1 -> Multiply3/2
  C_X_C_Y_C_Z/1 -> Selector4/1
  Constant/1 -> Minus/1
  Constant1/1 -> Minus/2
  Constant2/1 -> Divide/1
  Minus/1 -> Divide1/1
  Constant3/1 -> Divide1/2
  Selector4/1 -> Multiply4/1
  Divide1/1 -> Multiply4/2
  Multiply4/1 -> Sum/5
  Multiply1/1 -> Sum/3
  Multiply3/1 -> Sum/2
  alpha_t/1 -> Radians to Degrees/1
  Radians to Degrees/1 -> 2-D Lookup Table1/2, 2-D Lookup Table/2
  Sum/1 -> C_M_A/1

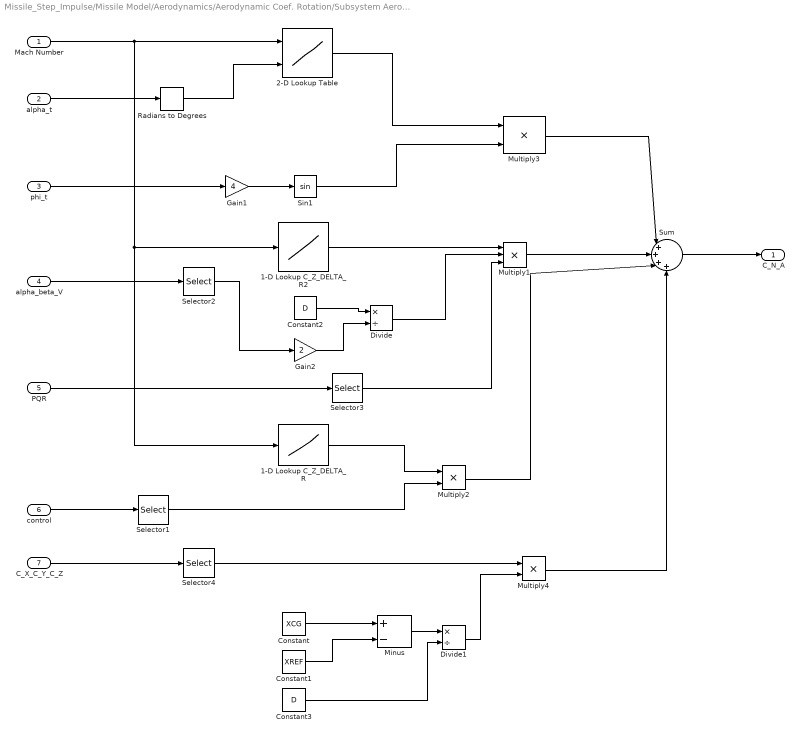
== system Missile_Step_Impulse/Missile Model/Aerodynamics/Aerodynamic Coef. Rotation/Subsystem Aero. Coef. Rotation/Subsystem C_N_A ==
  Mach Number : Inport
  alpha_t : Inport  Port=2
  phi_t : Inport  Port=3
  alpha_beta_V : Inport  Port=4
  PQR : Inport  Port=5
  control : Inport  Port=6
  C_X_C_Y_C_Z : Inport  Port=7
  1-D Lookup C_Z_DELTA_R : Lookup_n-D  NumberOfTableDimensions=1  BreakpointsForDimension1=Tbl_MACH  Table=Tbl_CN_DEL_Y  InternalRulePriority=Speed  RndMeth=Simplest  InputSameDT=on
  1-D Lookup C_Z_DELTA_R2 : Lookup_n-D  NumberOfTableDimensions=1  BreakpointsForDimension1=Tbl_MACH  Table=Tbl_CN_R  InternalRulePriority=Speed  RndMeth=Simplest  InputSameDT=on
  2-D Lookup Table : Lookup_n-D  BreakpointsForDimension1=Tbl_MACH  BreakpointsForDimension2=Tbl_ALPHAT  Table=Tbl_CN_PHIT  InternalRulePriority=Speed  RndMeth=Simplest  InputSameDT=on
  Constant : Constant  Value=XCG
  Constant1 : Constant  Value=XREF
  Constant2 : Constant  Value=D
  Constant3 : Constant  Value=D
  Divide : Product  Inputs=*/
  Divide1 : Product  Inputs=*/
  Gain1 : Gain  Gain=4
  Gain2 : Gain  Gain=2
  Minus : Sum  Inputs=+-
  Multiply1 : Product  Inputs=3
  Multiply2 : Product
  Multiply3 : Product
  Multiply4 : Product
  Radians to Degrees : simulink_extras/Transformations/Radians to Degrees
  Selector1 : Selector  InputPortWidth=3  IndexOptions=Index vector (dialog)  Indices=[3]  OutputSizes=1
  Selector2 : Selector  InputPortWidth=3  IndexOptions=Index vector (dialog)  Indices=[3]  OutputSizes=1
  Selector3 : Selector  InputPortWidth=3  IndexOptions=Index vector (dialog)  Indices=[3]  OutputSizes=1
  Selector4 : Selector  InputPortWidth=3  IndexOptions=Index vector (dialog)  Indices=[2]  OutputSizes=1
  Sin1 : Trigonometry
  Sum : Sum  Inputs=|++++
  C_N_A : Outport
  wires:
  2-D Lookup Table/1 -> Multiply3/1
  alpha_t/1 -> Radians to Degrees/1
  Sum/1 -> C_N_A/1
  Mach Number/1 -> 2-D Lookup Table/1, 1-D Lookup C_Z_DELTA_R/1, 1-D Lookup C_Z_DELTA_R2/1
  1-D Lookup C_Z_DELTA_R2/1 -> Multiply1/1
  1-D Lookup C_Z_DELTA_R/1 -> Multiply2/1
  Multiply2/1 -> Sum/3
  Sin1/1 -> Multiply3/2
  phi_t/1 -> Gain1/1
  Gain1/1 -> Sin1/1
  alpha_beta_V/1 -> Selector2/1
  Selector2/1 -> Gain2/1
  Divide/1 -> Multiply1/2
  PQR/1 -> Selector3/1
  Selector3/1 -> Multiply1/3
  control/1 -> Selector1/1
  Selector1/1 -> Multiply2/2
  C_X_C_Y_C_Z/1 -> Selector4/1
  Constant/1 -> Minus/1
  Constant1/1 -> Minus/2
  Constant2/1 -> Divide/1
  Minus/1 -> Divide1/1
  Constant3/1 -> Divide1/2
  Selector4/1 -> Multiply4/1
  Divide1/1 -> Multiply4/2
  Multiply4/1 -> Sum/4
  Multiply1/1 -> Sum/2
  Multiply3/1 -> Sum/1
  Radians to Degrees/1 -> 2-D Lookup Table/2
  Gain2/1 -> Divide/2

== system Missile_Step_Impulse/Missile Model/Aerodynamics/Aerodynamic Coef. Translation/Subsystem Aero. Coef. Translation/Subsystem C_X_A ==
  Mach Number : Inport
  alpha_t : Inport  Port=2
  delta_eff : Inport  Port=3
  1-D Lookup C_X_0 : Lookup_n-D  NumberOfTableDimensions=1  BreakpointsForDimension1=Tbl_MACH  Table=Tbl_CX_0  DiagnosticForOutOfRangeInput=Warning  InternalRulePriority=Speed  RndMeth=Simplest  InputSameDT=on
  1-D Lookup C_X_ALPHA_T : Lookup_n-D  NumberOfTableDimensions=1  BreakpointsForDimension1=Tbl_MACH  BeginIndexSearchUsingPreviousIndexResult=on  Table=Tbl_CX_ALPHAT  DiagnosticForOutOfRangeInput=Warning  InternalRulePriority=Speed  RndMeth=Simplest  InputSameDT=on
  1-D Lookup C_X_DELTA_EFF : Lookup_n-D  NumberOfTableDimensions=1  BreakpointsForDimension1=Tbl_MACH  Table=Tbl_CX_DEL_EFF  DiagnosticForOutOfRangeInput=Warning  InternalRulePriority=Speed  RndMeth=Simplest  InputSameDT=on
  Display : Display
  Multiply : Product
  Multiply1 : Product
  Scope : Scope
  Square : Math  Operator=square  SaturateOnIntegerOverflow=on
  Sum : Sum  Inputs=|+++
  C_X_A : Outport
  wires:
  Multiply/1 -> Sum/2
  Multiply1/1 -> Display/1, Sum/3
  1-D Lookup C_X_DELTA_EFF/1 -> Multiply1/1
  1-D Lookup C_X_ALPHA_T/1 -> Multiply/1
  1-D Lookup C_X_0/1 -> Sum/1
  Mach Number/1 -> 1-D Lookup C_X_DELTA_EFF/1, 1-D Lookup C_X_ALPHA_T/1, Scope/1, 1-D Lookup C_X_0/1
  Sum/1 -> C_X_A/1
  alpha_t/1 -> Multiply/2
  delta_eff/1 -> Square/1
  Square/1 -> Multiply1/2

== system Missile_Step_Impulse/Missile Model/Aerodynamics/Aerodynamic Coef. Translation/Subsystem Aero. Coef. Translation/Subsystem C_Y_A ==
  Mach Number : Inport
  alpha_t : Inport  Port=2
  control : Inport  Port=3
  phi_t : Inport  Port=4
  1-D Lookup C_Y_DELTA_Y : Lookup_n-D  NumberOfTableDimensions=1  BreakpointsForDimension1=Tbl_MACH  Table=Tbl_CY_DEL_Y  DiagnosticForOutOfRangeInput=Warning  InternalRulePriority=Speed  RndMeth=Simplest  InputSameDT=on
  2-D Lookup CY_PHIT : Lookup_n-D  BreakpointsForDimension1=Tbl_MACH  BreakpointsForDimension2=Tbl_ALPHAT  Table=Tbl_CY_PHIT  DiagnosticForOutOfRangeInput=Warning  InternalRulePriority=Speed  RndMeth=Simplest  InputSameDT=on
  Gain : Gain  Gain=4
  Multiply1 : Product
  Multiply2 : Product
  Radians to Degrees : simulink_extras/Transformations/Radians to Degrees
  Sin : Trigonometry
  Sum : Sum  Inputs=|++
  delta_y : Selector  InputPortWidth=3  IndexOptions=Index vector (dialog)  Indices=[3]  OutputSizes=1
  C_Y_A : Outport
  wires:
  Multiply1/1 -> Sum/2
  1-D Lookup C_Y_DELTA_Y/1 -> Multiply1/1
  2-D Lookup CY_PHIT/1 -> Multiply2/1
  Mach Number/1 -> 1-D Lookup C_Y_DELTA_Y/1, 2-D Lookup CY_PHIT/1
  Sum/1 -> C_Y_A/1
  Gain/1 -> Sin/1
  phi_t/1 -> Gain/1
  control/1 -> delta_y/1
  alpha_t/1 -> Radians to Degrees/1
  delta_y/1 -> Multiply1/2
  Sin/1 -> Multiply2/2
  Multiply2/1 -> Sum/1
  Radians to Degrees/1 -> 2-D Lookup CY_PHIT/2

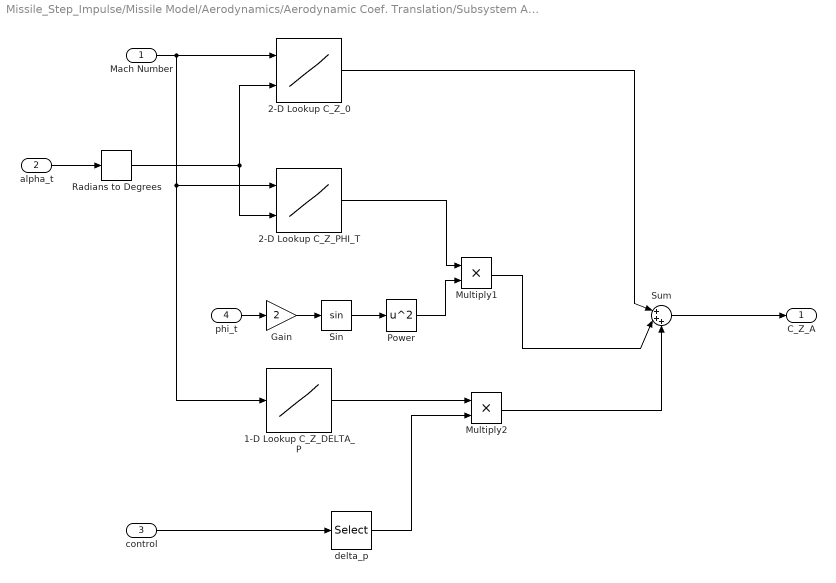
== system Missile_Step_Impulse/Missile Model/Aerodynamics/Aerodynamic Coef. Translation/Subsystem Aero. Coef. Translation/Subsystem C_Z_A ==
  Mach Number : Inport
  alpha_t : Inport  Port=2
  control : Inport  Port=3
  phi_t : Inport  Port=4
  1-D Lookup C_Z_DELTA_P : Lookup_n-D  NumberOfTableDimensions=1  BreakpointsForDimension1=Tbl_MACH  Table=Tbl_CZ_DEL_P  InternalRulePriority=Speed  RndMeth=Simplest  InputSameDT=on
  2-D Lookup C_Z_0 : Lookup_n-D  BreakpointsForDimension1=Tbl_MACH  BreakpointsForDimension2=Tbl_ALPHAT  Table=Tbl_CZ_0  DiagnosticForOutOfRangeInput=Warning  InternalRulePriority=Speed  RndMeth=Simplest  InputSameDT=on
  2-D Lookup C_Z_PHI_T : Lookup_n-D  BreakpointsForDimension1=Tbl_MACH  BreakpointsForDimension2=Tbl_ALPHAT  Table=Tbl_CZ_PHIT  InternalRulePriority=Speed  RndMeth=Simplest  InputSameDT=on
  Gain : Gain  Gain=2
  Multiply1 : Product
  Multiply2 : Product
  Power : Math  Operator=square  SaturateOnIntegerOverflow=on
  Radians to Degrees : simulink_extras/Transformations/Radians to Degrees
  Sin : Trigonometry
  Sum : Sum  Inputs=|+++
  delta_p : Selector  InputPortWidth=3  IndexOptions=Index vector (dialog)  Indices=[2]  OutputSizes=1
  C_Z_A : Outport
  wires:
  2-D Lookup C_Z_0/1 -> Sum/1
  delta_p/1 -> Multiply2/2
  alpha_t/1 -> Radians to Degrees/1
  control/1 -> delta_p/1
  Sum/1 -> C_Z_A/1
  Mach Number/1 -> 2-D Lookup C_Z_PHI_T/1, 1-D Lookup C_Z_DELTA_P/1, 2-D Lookup C_Z_0/1
  2-D Lookup C_Z_PHI_T/1 -> Multiply1/1
  Multiply1/1 -> Sum/2
  Gain/1 -> Sin/1
  phi_t/1 -> Gain/1
  Sin/1 -> Power/1
  Power/1 -> Multiply1/2
  1-D Lookup C_Z_DELTA_P/1 -> Multiply2/1
  Multiply2/1 -> Sum/3
  Radians to Degrees/1 -> 2-D Lookup C_Z_0/2, 2-D Lookup C_Z_PHI_T/2
